simulink model "sampleModel1598_1_sub_sub"  (R2023a)
settings: Solver=VariableStepAuto  StartTime=0.0  StopTime=10.0  RelTol=1e-3
libraries: hdlsllib x4, simulink x3
settings Model: Creator=user1  LastModifiedBy=user1
settings OptimizationCC: BlockReduction=off  ConditionallyExecuteInputs=off

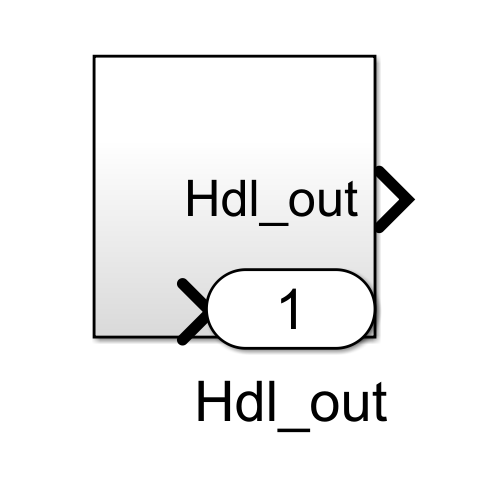
[thumbnail: Simulink's stored preview of the top-level diagram]
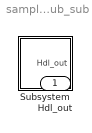
== system sampleModel1598_1_sub_sub ==
  Subsystem : Subsystem
  Hdl_out : Outport  OutDataTypeStr=uint8

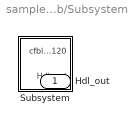
== system sampleModel1598_1_sub_sub/Subsystem ==
  Subsystem : Subsystem
  Hdl_out : Outport  OutDataTypeStr=uint8

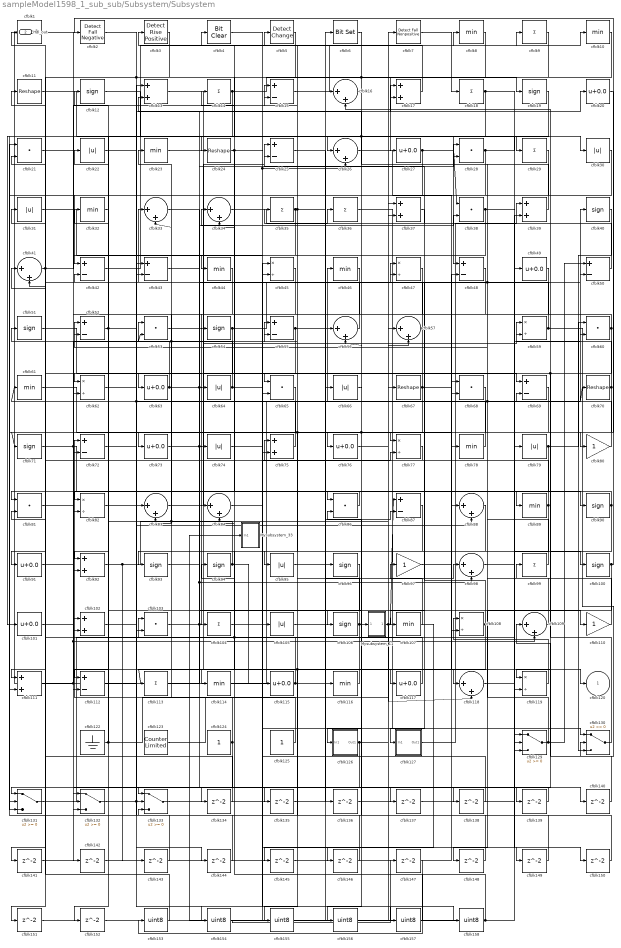
== system sampleModel1598_1_sub_sub/Subsystem/Subsystem ==
  Mysubsystem_11 : Subsystem  TreatAsAtomicUnit=on  RTWFcnName=Mysubsystem_11
      settings: RTWFcnNameOpts=User specified  RTWFileNameOpts=Use function name
  Mysubsystem_33 : Subsystem  TreatAsAtomicUnit=on  RTWFcnName=Mysubsystem_33
      settings: RTWFcnNameOpts=User specified  RTWFileNameOpts=Use function name
  cfblk1 : ArithShift  BitShiftNumber=8
  cfblk{8,10,23,32,44,46,61,78,89,107,114,116} (12 alike) : MinMax  OutDataTypeStr=uint8
  cfblk{12,19,40,51,54,71,90,93..94,96,100,106} (12 alike) : Signum
  cfblk{20,27,49,63,73,76,91,101,115,117} (10 alike) : Bias  Bias=0.0  SaturateOnIntegerOverflow=off
  cfblk{13,17,37,39,75,92,102,111} (8 alike) : Sum  OutDataTypeStr=uint8
  cfblk{21,28,38,53,60,65,68,81,86,103} (10 alike) : DotProduct  OutDataTypeStr=uint8
  cfblk{9,14,18,29,35..36,99,104,113} (9 alike) : Sum  Inputs=+  OutDataTypeStr=uint8
  cfblk{22,30..31,64,66,74,79,95,105} (9 alike) : Abs  OutDataTypeStr=uint8  SaturateOnIntegerOverflow=off
  cfblk{45,47,59,62,77,82,108,119} (8 alike) : Product  Inputs=*/  OutDataTypeStr=uint8  RndMeth=Zero  SaturateOnIntegerOverflow=on
  cfblk{16,26,33..34,41,56..57,83..84,88,98,109,118} (13 alike) : Sum  Inputs=|++  OutDataTypeStr=uint8
  cfblk{11,24,67,70} (4 alike) : Reshape
  cfblk110 : Gain  OutDataTypeStr=uint8
  cfblk{15,25,42..43,48,50,52,55,69,72,87,112} (12 alike) : Sum  Inputs=+-  OutDataTypeStr=uint8
  cfblk122 : Ground
  cfblk123 : hdlsllib/Sources/Counter Limited  uplimit=7  tsamp=-1
  cfblk124 : Constant  OutDataTypeStr=uint8  SampleTime=-1
  cfblk125 : Constant  OutDataTypeStr=uint8  SampleTime=-1
  cfblk126 : Subsystem
      settings: LibrarySourceBlock=|
      | hdlsllib/Ports &
      | Subsystems/Subsystem
  cfblk127 : Subsystem
      settings: LibrarySourceBlock=|
      | hdlsllib/Ports &
      | Subsystems/Subsystem
  cfblk{129..133} (5 alike) : Switch  OutDataTypeStr=uint8  SaturateOnIntegerOverflow=off  InputSameDT=off
  cfblk{134..152} (19 alike) : Delay  SampleTime=1
  cfblk{153..158} (6 alike) : DataTypeConversion  OutDataTypeStr=uint8  SaturateOnIntegerOverflow=off  RndMeth=Floor
  cfblk2 : hdlsllib/Logic and Bit Operations/Detect Fall Negative  vinit=0  OutDataTypeStr=uint8
  cfblk3 : hdlsllib/Logic and Bit Operations/Detect Rise Positive  vinit=0  OutDataTypeStr=uint8
  cfblk4 : simulink/Logic and Bit Operations/Bit Clear  iBit=0
      settings: LibrarySourceBlock=|
      | hdlsllib/Logic and Bit
      | Operations/Bit Clear
  cfblk5 : simulink/Logic and Bit Operations/Detect Change  vinit=0  OutDataTypeStr=uint8
      settings: LibrarySourceBlock=|
      | hdlsllib/Logic and Bit
      | Operations/Detect
      | Change
  cfblk6 : simulink/Logic and Bit Operations/Bit Set  iBit=0
      settings: LibrarySourceBlock=|
      | hdlsllib/Logic and Bit
      | Operations/Bit Set
  cfblk7 : hdlsllib/Logic and Bit Operations/Detect Fall Nonpositive  vinit=0  OutDataTypeStr=uint8
  cfblk80 : Gain  OutDataTypeStr=uint8
  cfblk97 : Gain  OutDataTypeStr=uint8
  cfblk120 : Outport  OutDataTypeStr=uint8  VectorParamsAs1DForOutWhenUnconnected=off
  Hdl_out : Outport  Port=2  OutDataTypeStr=uint8
  wires:
  Mysubsystem_11/1(Out1) -> cfblk145/1
  cfblk158/1 -> Mysubsystem_33/1(In1), cfblk14/1
  cfblk157/1 -> cfblk4/1
  cfblk82/1 -> cfblk157/1
  cfblk156/1 -> cfblk49/1
  cfblk6/1 -> cfblk156/1
  cfblk155/1 -> cfblk6/1
  cfblk154/1 -> cfblk147/1
  cfblk2/1 -> cfblk154/1
  cfblk153/1 -> cfblk1/1
  cfblk147/1 -> cfblk153/1
  cfblk152/1 -> cfblk67/1
  cfblk96/1 -> cfblk152/1
  cfblk151/1 -> cfblk75/2
  cfblk150/1 -> cfblk84/2
  cfblk149/1 -> cfblk15/2
  cfblk74/1 -> cfblk149/1
  cfblk148/1 -> cfblk86/2
  cfblk146/1 -> cfblk133/3
  cfblk47/1 -> cfblk146/1
  cfblk145/1 -> cfblk56/1
  cfblk144/1 -> cfblk21/1
  cfblk143/1 -> cfblk13/1
  cfblk142/1 -> cfblk48/2
  cfblk91/1 -> cfblk142/1
  cfblk141/1 -> cfblk37/2
  cfblk3/1 -> cfblk141/1
  cfblk140/1 -> cfblk109/1
  cfblk139/1 -> cfblk131/1
  cfblk138/1 -> cfblk45/1
  cfblk112/1 -> cfblk138/1
  cfblk137/1 -> cfblk39/2
  cfblk136/1 -> cfblk68/1
  cfblk25/1 -> cfblk136/1
  cfblk135/1 -> cfblk16/1
  cfblk93/1 -> cfblk135/1
  cfblk134/1 -> cfblk41/1
  cfblk101/1 -> cfblk134/1
  cfblk88/1 -> cfblk93/1
  cfblk69/1 -> cfblk84/1
  cfblk37/1 -> cfblk127/1(In1)
  cfblk65/1 -> cfblk112/1
  cfblk21/1 -> cfblk132/1
  cfblk68/1 -> cfblk126/1(In1), cfblk71/1
  cfblk12/1 -> cfblk26/1
  cfblk18/1 -> cfblk129/1, cfblk131/2
  cfblk75/1 -> cfblk41/2
  cfblk103/1 -> cfblk38/2
  cfblk10/1 -> cfblk56/2, cfblk24/1
  cfblk1/1 -> cfblk120/1, cfblk109/2
  cfblk97/1 -> cfblk69/2
  cfblk64/1 -> cfblk105/1, cfblk31/1
  cfblk43/1 -> cfblk108/2, cfblk98/2
  cfblk77/1 -> cfblk72/2
  cfblk70/1 -> cfblk59/2, cfblk131/3
  cfblk27/1 -> cfblk38/1, cfblk62/2
  cfblk57/1 -> cfblk21/2, cfblk92/2
  cfblk84/1 -> cfblk77/2
  cfblk5/1 -> cfblk43/2
  cfblk105/1 -> cfblk98/1
  cfblk90/1 -> cfblk119/1, cfblk86/1
  cfblk89/1 -> cfblk107/1, cfblk51/1
  cfblk45/1 -> cfblk65/2
  cfblk123/1 -> cfblk66/1
  cfblk119/1 -> cfblk108/1
  cfblk131/1 -> cfblk60/2
  cfblk40/1 -> cfblk130/3
  cfblk24/1 -> cfblk26/2, cfblk129/3, cfblk74/1
  cfblk130/1 -> cfblk16/2
  cfblk48/1 -> cfblk92/1
  cfblk87/1 -> cfblk114/1
  cfblk115/1 -> cfblk81/2, cfblk87/2, Hdl_out/1
  cfblk33/1 -> cfblk90/1
  cfblk76/1 -> cfblk10/1
  cfblk80/1 -> cfblk34/1
  cfblk118/1 -> cfblk79/1
  cfblk79/1 -> cfblk60/1, cfblk129/2
  cfblk30/1 -> cfblk103/2
  cfblk81/1 -> cfblk102/1
  cfblk102/1 -> cfblk43/1
  cfblk28/1 -> cfblk30/1, cfblk111/2
  cfblk83/1 -> cfblk57/2
  cfblk49/1 -> cfblk82/2
  cfblk71/1 -> cfblk116/1, cfblk53/1, cfblk89/1
  cfblk11/1 -> cfblk29/1
  cfblk51/1 -> cfblk64/1
  cfblk61/1 -> cfblk88/1
  cfblk31/1 -> cfblk44/1
  cfblk60/1 -> cfblk111/1, cfblk139/1, cfblk54/1
  cfblk132/1 -> cfblk88/2, cfblk144/1
  cfblk7/1 -> cfblk18/1
  cfblk98/1 -> cfblk100/1
  cfblk20/1 -> cfblk80/1
  cfblk92/1 -> cfblk7/1, cfblk143/1
  cfblk46/1 -> cfblk104/1
  cfblk22/1 -> cfblk45/2
  cfblk99/1 -> cfblk75/1
  cfblk4/1 -> cfblk158/1
  cfblk111/1 -> cfblk55/1, cfblk140/1
  cfblk56/1 -> cfblk33/1
  cfblk72/1 -> cfblk70/1, cfblk20/1
  cfblk133/1 -> cfblk68/2
  cfblk129/1 -> cfblk61/1, cfblk52/2, cfblk50/1
  cfblk16/1 -> cfblk76/1
  cfblk8/1 -> cfblk27/1
  cfblk13/1 -> cfblk69/1
  cfblk113/1 -> Mysubsystem_11/1(In1), cfblk17/2
  cfblk9/1 -> cfblk133/2, cfblk112/2
  cfblk23/1 -> cfblk77/1
  cfblk26/1 -> cfblk78/1
  cfblk107/1 -> cfblk97/1
  cfblk35/1 -> cfblk5/1, cfblk118/1, cfblk132/2
  cfblk41/1 -> cfblk15/1, cfblk151/1
  cfblk108/1 -> cfblk113/1, cfblk155/1, cfblk47/1
  cfblk117/1 -> cfblk103/1
  cfblk110/1 -> cfblk35/1
  cfblk34/1 -> cfblk36/1
  cfblk114/1 -> cfblk40/1
  cfblk14/1 -> cfblk19/1, cfblk62/1
  cfblk53/1 -> cfblk117/1
  cfblk116/1 -> cfblk11/1, cfblk94/1
  cfblk52/1 -> cfblk22/1, cfblk137/1
  cfblk78/1 -> cfblk46/1
  cfblk109/1 -> cfblk99/1
  cfblk62/1 -> cfblk83/1
  cfblk19/1 -> cfblk48/1
  cfblk122/1 -> cfblk57/1, cfblk52/1
  cfblk17/1 -> cfblk3/1
  cfblk106/1 -> cfblk87/1, cfblk118/2, cfblk102/2, cfblk55/2
  cfblk94/1 -> cfblk23/1, cfblk12/1, cfblk115/1
  cfblk126/1(Out1) -> cfblk37/1, cfblk132/3
  cfblk73/1 -> cfblk59/1, cfblk47/2
  cfblk55/1 -> cfblk65/1, cfblk17/1
  cfblk100/1 -> cfblk2/1, cfblk148/1
  cfblk127/1(Out1) -> cfblk39/1
  cfblk66/1 -> cfblk106/1
  cfblk95/1 -> cfblk96/1
  cfblk38/1 -> cfblk82/1, cfblk150/1
  cfblk44/1 -> cfblk73/1
  cfblk125/1 -> cfblk72/1
  cfblk63/1 -> cfblk25/2, cfblk28/1, cfblk32/1
  cfblk42/1 -> cfblk8/1
  cfblk59/1 -> cfblk28/2, cfblk34/2, cfblk130/2
  cfblk32/1 -> cfblk42/2
  cfblk54/1 -> cfblk91/1, cfblk50/2
  cfblk15/1 -> cfblk9/1
  cfblk67/1 -> cfblk95/1, cfblk83/2, cfblk63/1, cfblk119/2
  cfblk104/1 -> cfblk110/1
  cfblk29/1 -> cfblk42/1
  cfblk39/1 -> cfblk101/1, cfblk13/2
  cfblk50/1 -> cfblk25/1
  cfblk36/1 -> cfblk130/1
  cfblk86/1 -> cfblk81/1
  cfblk124/1 -> cfblk33/2, cfblk53/2, cfblk133/1

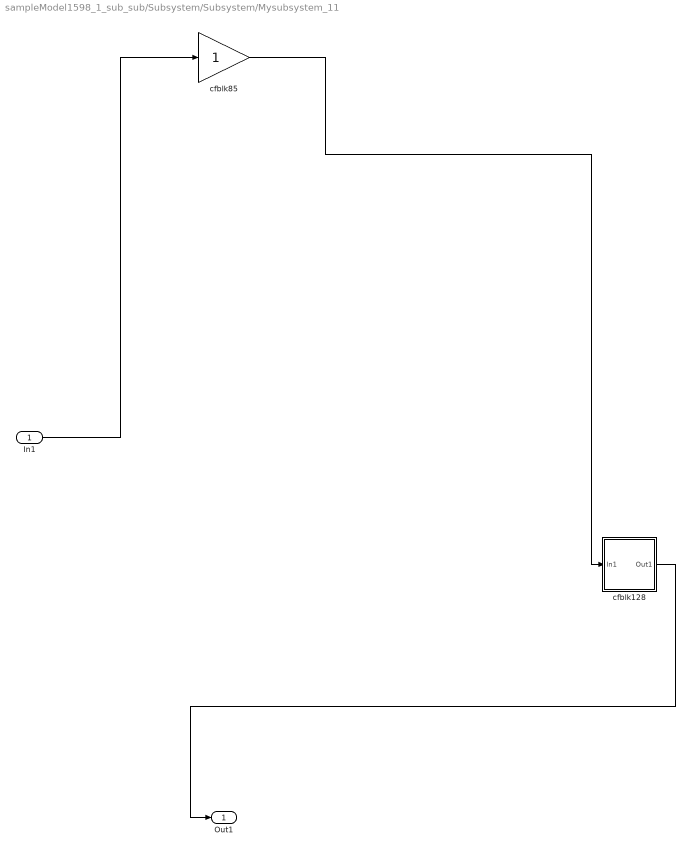
== system sampleModel1598_1_sub_sub/Subsystem/Subsystem/Mysubsystem_11 ==
  In1 : Inport
  cfblk128 : Subsystem
      settings: LibrarySourceBlock=|
      | hdlsllib/Ports &
      | Subsystems/Subsystem
  cfblk85 : Gain
  Out1 : Outport
  wires:
  cfblk85/1 -> cfblk128/1(In1)
  In1/1 -> cfblk85/1
  cfblk128/1(Out1) -> Out1/1

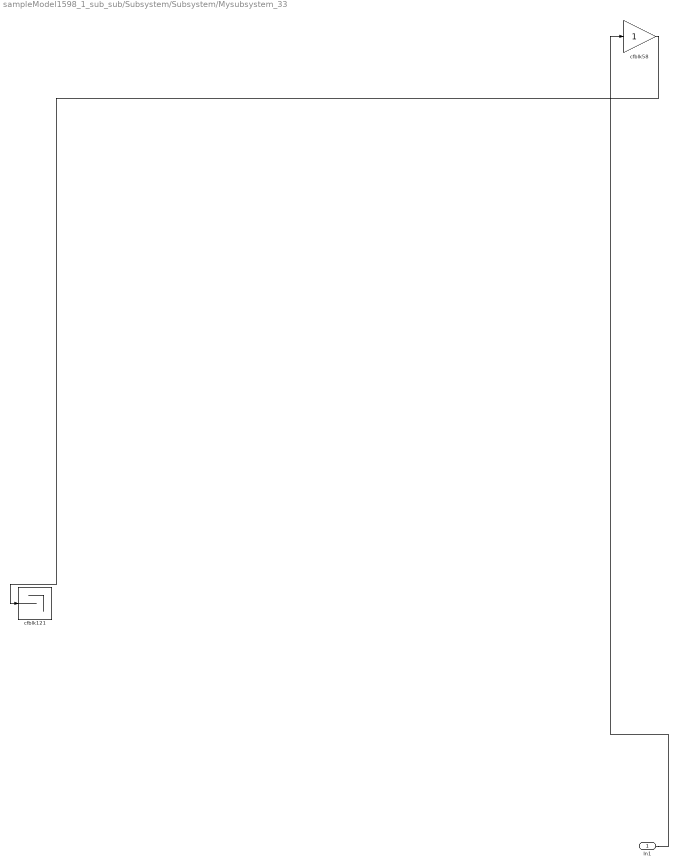
== system sampleModel1598_1_sub_sub/Subsystem/Subsystem/Mysubsystem_33 ==
  In1 : Inport
  cfblk121 : Terminator
  cfblk58 : Gain
  wires:
  cfblk58/1 -> cfblk121/1
  In1/1 -> cfblk58/1

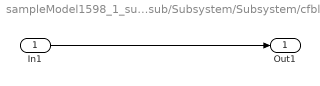
== system sampleModel1598_1_sub_sub/Subsystem/Subsystem/cfblk126 ==
  In1 : Inport
  Out1 : Outport
  wires:
  In1/1 -> Out1/1

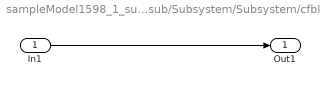
== system sampleModel1598_1_sub_sub/Subsystem/Subsystem/cfblk127 ==
  In1 : Inport
  Out1 : Outport
  wires:
  In1/1 -> Out1/1

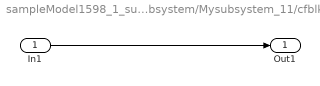
== system sampleModel1598_1_sub_sub/Subsystem/Subsystem/Mysubsystem_11/cfblk128 ==
  In1 : Inport
  Out1 : Outport
  wires:
  In1/1 -> Out1/1
